simulink model "MassflowModel"  (R2020b)
settings: Solver=VariableStepAuto  StartTime=0.0  StopTime=55.357742309570312  RelTol=1e-3  AbsTol=1e-3
values from neighbouring files (symbols this model uses):
  coil_specific_heat_transfer = 20    [LoadDataForParameterEstimation.m]
  coil_voltage = 20    [LoadDataForParameterEstimation.m]
libraries: fl_lib x13, nesl_utility x10, SimscapeFluids_lib x1, SignalEditorBlockLib x1
(part 3 of 3)

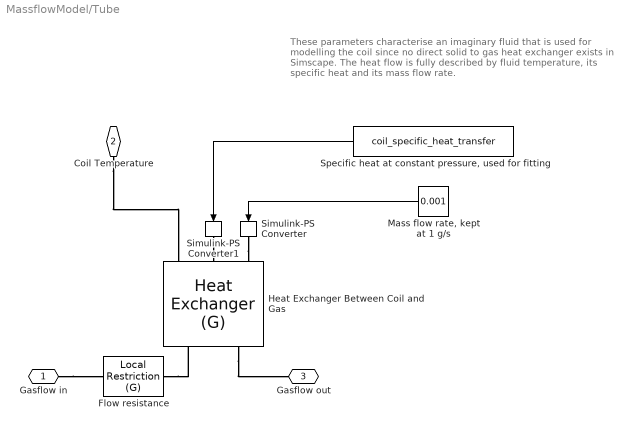
== system MassflowModel/Tube ==
  note: These parameters characterise an imaginary
      | fluid that is used for modelling the coil since no direct
      | solid to gas heat exchanger exists in Simscape.
      | The heat flow is fully described by fluid
      | temperature, its specific heat and its mass flow rate.
  Flow resistance : fl_lib/Gas/Elements/Local Restriction (G)  restriction_type=foundation.enum.restriction_type.fixed  restriction_area=0.0011 m^2  min_area=1e-10 m^2  max_area=0.005 m^2  area=0.00126 m^2  Cd=0.64  B_lam=0.999
      settings: SourceProductBaseCode=SS  InternalSimscapePortConfiguration="{\"Bottom\":[],\"Left\":[{\"id\":\"A\",\"label\":\"A\",\"type\":\"foundation.gas.gas\"}],\"Right\":[{\"id\":\"B\",\"label\":\"B\",\"type\":\"foundation.gas.gas\"}],\"Top\":[]}"
  Heat Exchanger Between Coil and Gas : SimscapeFluids_lib/Fluid Network Interfaces/Heat Exchangers/Heat Exchanger (G)  hex_type=fluids.interfaces.enum.flow_arrangement_spec.parallel_counter  cross_type=fluids.interfaces.enum.cross_flow_heat_exchanger_G_spec.mixed_mixed  shell_num=1  NTU_TLU=[.5, 1, 2, 3, 4, 5]  CR_TLU=[0, .25, .5, .75, 1]  eff_TLU=[.3, .3, .3, .3, .3; .6, .55, .5, .47, .43; .85, .76, .68, .61, .55; .94, .83, .72, .65, .58; .98, .86, .75, .66, .58; .99, .86, .75, .66, .58]  R_wall=1.6e-4 K/W  min_flow_area_1=0.01 m^2  Dh_press_1=0.1 m  gas_volume_1=0.01 m^3  Re_lam_1=2000  Re_tur_1=4000  pressure_loss_spec_1=fluids.interfaces.enum.pressure_loss_spec.constant  heat_transfer_area_2=0.4 m^2  fouling_factor_2=1e-4 m^2*K/W  min_heat_coeff_2=5 W/(m^2 * K)  pressure_loss_coeff_1=0.1  length_press_1=1 m  length_add_1=0.1 m  roughness_1=15e-6 m  Re_friction_TLU_1=[400, 1000, 1500, 3000, 4000, 6000, 10000, 20000, 40000, 60000, 100000, 100000000]  friction_factor_TLU_1=[.264, .112, .071, .0417, .0387, .0268, .025, .0232, .0226, .022, .0214, .0214]  shape_factor_1=64  Re_Euler_TLU_1=[50, 500, 1000, 2000]  Euler_TLU_1=[4.4505, .6864, .4791, .3755]  heat_transfer_spec_1=fluids.interfaces.enum.heat_transfer_spec.constant  heat_coeff_1=100 W/(m^2 * K)  length_heat_1=1 m  Nu_lam_1=3.66  Re_Colburn_TLU_1=[100, 150, 1000]  Colburn_factor_TLU_1=[.019, .013, .002]  Re_Nu_TLU_1=[100, 150, 1000]  Pr_Nu_TLU_1=[1, 10]  Nu_TLU_1=[3.72, 4.21; 3.75, 4.44; 4.21, 7.15]  heat_transfer_area_1=0.4 m^2  fouling_factor_1=1e-4 m^2*K/W  mdot_threshold_1=1e-6 kg/s  min_heat_coeff_1=5 W/(m^2 * K)  T0_1=25 degC  p0_1=0.101325 MPa  mdot1_TLU=[.3, .5, .6, .7, 1, 1.4, 1.9, 2.3] kg/s  mdot2_TLU=[.3, .5, 1, 1.3, 1.7, 2, 2.6, 3.3] kg/s  SD_TLU=[.324, .3533, .404, .4253, .4333, .4373, .4453, .4533; .3813, .424, .496, .5307, .544, .5547, .5693, .5787; .4267, .4827, .5813, .6173, .6413, .6573, .672, .6827; .4613, .528, .64, .6987, .7267, .7467, .7707, .7853; .5533, .6467, .8227, .928, .9853, 1.0187, 1.0653, 1.0973; .58, .688, .8853, 1.0147, 1.08, 1.124, 1.176, 1.2147; .624, .7467, .992, 1.148, 1.244, 1.304, 1.3773, 1.4267; .656, .7907, 1.0667, 1.26, 1.376, 1.452, 1.548, 1.612] kW/K  Q_check=fluids.interfaces.enum.SD_max_check.none  mdot_dp_TLU_1=[.3, .5, 1, 1.5, 2, 2.5] kg/s  p_diff_TLU_1=[3, 5, 10, 25, 35, 50] * 1e-3 MPa  T_ref_in_1=293.15 K  p_ref_in_1=0.101325 MPa  area_1=0.01 m^2
      settings: SourceProductBaseCode=SH  InternalSimscapePortConfiguration="{\"Bottom\":[],\"Left\":[{\"id\":\"A1\",\"label\":\"A1\",\"type\":\"foundation.gas.gas\"},{\"id\":\"B1\",\"label\":\"B1\",\"type\":\"foundation.gas.gas\"}],\"Right\":[{\"id\":\"H2\",\"label\":\"H2\",\"type\":\"foundation.thermal.thermal\"},{\"id\":\"CP2\",\"label\":\"CP2\",\"type\":\"input\"},{\"id\":\"M2\",\"label\":\"M2\",\"type\":\"input\"}],\"Top\":[]}"
  "Mass flow rate, kept at 1 g/s" : Constant  Value=0.001
  Simulink-PS Converter : nesl_utility/Simulink-PS Converter  PhysicalDomain=network_engine_domain  SubClassName=ps_input  LeftPortType=input  RightPortType=output  PseudoPeriodic=off  Frequencies=[]  NoiseDistribution=none  NoiseParameters=[]  Unit=1  AffineConversion=off  FilteringAndDerivatives=provide  SimscapeFilterOrder=1  InputFilterTimeConstant=0.001  UdotUserProvided=0
  Simulink-PS Converter1 : nesl_utility/Simulink-PS Converter  PhysicalDomain=network_engine_domain  SubClassName=ps_input  LeftPortType=input  RightPortType=output  PseudoPeriodic=off  Frequencies=[]  NoiseDistribution=none  NoiseParameters=[]  Unit=1  AffineConversion=off  FilteringAndDerivatives=provide  SimscapeFilterOrder=1  InputFilterTimeConstant=0.001  UdotUserProvided=0
  "Specific heat at constant pressure, used for fitting" : Constant  Value=coil_specific_heat_transfer
  Gasflow in : PMIOPort  Side=Left
  Coil Temperature : PMIOPort  Port=2  Side=Right
  Gasflow out : PMIOPort  Port=3  Side=Right
  wires:
  "Specific heat at constant pressure, used for fitting"/1 -> Simulink-PS Converter1/1
  "Mass flow rate, kept at 1 g/s"/1 -> Simulink-PS Converter/1
  connections:
  Simulink-PS Converter/RConn1 -- Heat Exchanger Between Coil and Gas/RConn3
  Flow resistance/RConn1 -- Heat Exchanger Between Coil and Gas/LConn1
  Gasflow in/RConn1 -- Flow resistance/LConn1
  Simulink-PS Converter1/RConn1 -- Heat Exchanger Between Coil and Gas/RConn2
  Heat Exchanger Between Coil and Gas/LConn2 -- Gasflow out/RConn1
  Coil Temperature/RConn1 -- Heat Exchanger Between Coil and Gas/RConn1

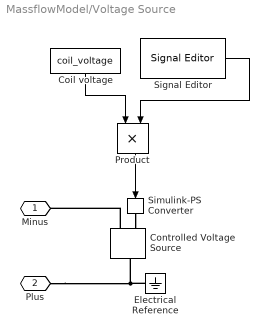
== system MassflowModel/Voltage Source ==
  Coil voltage : Constant  Value=coil_voltage
  Controlled Voltage Source : fl_lib/Electrical/Electrical Sources/Controlled Voltage Source
  Electrical Reference : fl_lib/Electrical/Electrical Elements/Electrical Reference
  Product : Product
  Signal Editor : SignalEditorBlockLib/Signal Editor  FileName=Scenario.mat  ActiveScenario=Scenario  ActiveSignal=PWM  IsBus=off  OutputBusObjectStr=Bus: BusObject  SampleTime=0  Interpolate=off  ZeroCross=off  OutputAfterFinalValue=Setting to zero  Unit=inherit  PreserveSignalName=on
  Simulink-PS Converter : nesl_utility/Simulink-PS Converter  PhysicalDomain=network_engine_domain  SubClassName=ps_input  LeftPortType=input  RightPortType=output  PseudoPeriodic=off  Frequencies=[]  NoiseDistribution=none  NoiseParameters=[]  Unit=1  AffineConversion=off  FilteringAndDerivatives=provide  SimscapeFilterOrder=1  InputFilterTimeConstant=0.001  UdotUserProvided=0
  Minus : PMIOPort  Side=Left
  Plus : PMIOPort  Port=2  Side=Left
  wires:
  Coil voltage/1 -> Product/1
  Product/1 -> Simulink-PS Converter/1
  Signal Editor/1 -> Product/2
  connections:
  Electrical Reference/LConn1 -- Plus/RConn1 -- Controlled Voltage Source/LConn1
  Simulink-PS Converter/RConn1 -- Controlled Voltage Source/RConn1
  Controlled Voltage Source/RConn2 -- Minus/RConn1

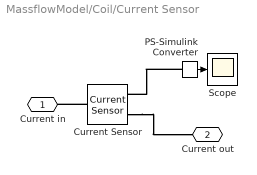
== system MassflowModel/Coil/Current Sensor ==
  Current Sensor : fl_lib/Electrical/Electrical Sensors/Current Sensor
  PS-Simulink Converter : nesl_utility/PS-Simulink Converter  PhysicalDomain=network_engine_domain  SubClassName=ps_output  LeftPortType=input  RightPortType=output  PseudoPeriodic=off  Frequencies=[]  Unit=inherit  AffineConversion=off
  Scope : Scope
  Current in : PMIOPort  Side=Left
  Current out : PMIOPort  Port=2  Side=Right
  wires:
  PS-Simulink Converter/1 -> Scope/1
  connections:
  PS-Simulink Converter/LConn1 -- Current Sensor/RConn1
  Current Sensor/RConn2 -- Current out/RConn1
  Current Sensor/LConn1 -- Current in/RConn1

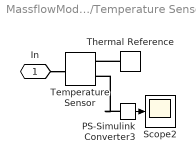
== system MassflowModel/Coil/Temperature Sensor ==
  PS-Simulink Converter3 : nesl_utility/PS-Simulink Converter  PhysicalDomain=network_engine_domain  SubClassName=ps_output  LeftPortType=input  RightPortType=output  PseudoPeriodic=off  Frequencies=[]  Unit=inherit  AffineConversion=off
  Scope2 : Scope
  Temperature Sensor : fl_lib/Thermal/Thermal Sensors/Temperature Sensor
  Thermal Reference : fl_lib/Thermal/Thermal Elements/Thermal Reference
  In : PMIOPort  Side=Right
  wires:
  PS-Simulink Converter3/1 -> Scope2/1
  connections:
  PS-Simulink Converter3/LConn1 -- Temperature Sensor/RConn2
  Thermal Reference/LConn1 -- Temperature Sensor/RConn1
  In/RConn1 -- Temperature Sensor/LConn1
